simulink library "breaker_lib"  (Simulink 8.1)
settings: Solver=ode45  StartTime=0.0  StopTime=10.0  RelTol=1e-3
values from neighbouring files (symbols this model uses):
  Ts = 100E-6    (= 0.0001)    [UnitTest_Breaker_init.m]
undefined symbols (not defined in the file): cb_mech_delay
libraries: powerlib x17, simulink x5, breaker_lib x4, powerlib_extras x2
settings Model: Creator=RE25624  LastModifiedBy=RE25624

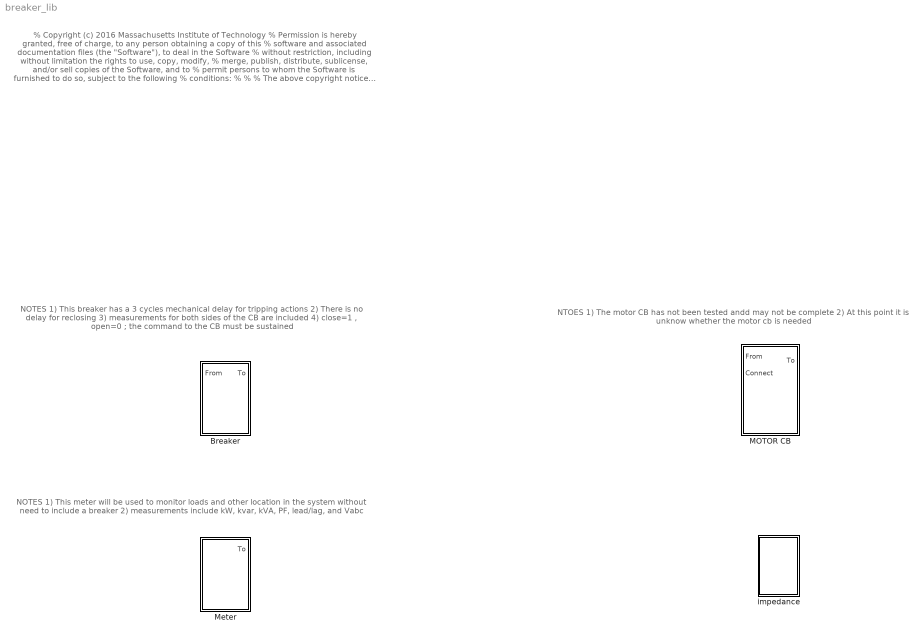
== system breaker_lib ==
  note: NTOES
      | 1) The motor CB has not been tested andd may not be complete
      | 2) At this point it is unknow whether the motor cb is needed
  note: NOTES
      | 1) This breaker has a 3 cycles mechanical delay for tripping actions
      | 2) There is no delay for reclosing
      | 3) measurements for both sides of the CB are included
      | 4) close=1 , open=0   ;  the command to the CB must be sustained
  note: NOTES
      | 1) This meter will be used to monitor loads and other location in the system without need to include a breaker
      | 2) measurements include kW, kvar, kVA, PF, lead/lag, and Vabc
  note: % Copyright (c) 2016 Massachusetts Institute of Technology
      | % Permission is hereby granted, free of charge, to any person obtaining a copy of this
      | % software and associated documentation files (the "Software"), to deal in the Software
      | % without restriction, including without limitation the rights to use, copy, modify,
      | % merge, publish, distribute, sublicense, and/or sell copies of the Software, and to
      | % permit persons to whom the Software is furnished to do so, subject to the following
      | % conditions:
      | %
      | %
      | % The above copyright notice and this permission notice shall be included in
      | % all copies or substantial portions of the Software.
      | %
      | % THE SOFTWARE IS PROVIDED "AS IS", WITHOUT WARRANTY OF ANY KIND, EXPRESS OR IMPLIED,
      | % INCLUDING BUT NOT LIMITED TO THE WARRANTIES OF MERCHANTABILITY, FITNESS FOR A
      | % PARTICULAR PURPOSE AND NONINFRINGEMENT. IN NO EVENT SHALL THE AUTHORS OR COPYRIGHT
      | % HOLDERS BE LIABLE FOR ANY CLAIM, DAMAGES OR OTHER LIABILITY, WHETHER IN AN ACTION
      | % OF CONTRACT, TORT OR OTHERWISE, ARISING FROM, OUT OF OR IN CONNECTION WITH THE
      | % SOFTWARE OR THE USE OR OTHER DEALINGS IN THE SOFTWARE.
      | %
      | %
      | %%
  Breaker : Subsystem  mask(Breaker){Ts=Ts, mech_delay=cb_mech_delay}
      mask prompts: Ts "Sampling Time [Sec]"; mech_delay "Open/Close Mechanical Delay [Sec]"
      mask help:
      | This block simulates the open/close behavior of a breaker. The logic (1-closed; 0-open) of operation is provided via external relay-blocks.
      | The breaker model also facilitates the system measurements for all logic functions to operate.
      | The connectivity convention adopted for this block is as follows: ABC indicates the “entry-point” or line, and the abc indicates the “exit-point” or bus.
      |
      | Ts [s]: simulation time step
      | Breaker mechanical open/close delay [s]
      mask init:
      | mech_delay = floor(mech_delay/Ts);
  MOTOR CB : Subsystem  mask(Breaker){Ts=Ts}
      mask prompts: Ts "Sampling Time [Sec]"
      mask help:
      | This block simulates the open/close behavior of a breaker. The logic (1-closed; 0-open) of operation is provided via external relay-blocks.
      | The breaker model also facilitates the system measurements for all logic functions to operate.
      | The connectivity convention adopted for this block is as follows: ABC indicates the “entry-point” or line, and the abc indicates the “exit-point” or bus.
  Meter : Subsystem  mask(Breaker){Ts=Ts}
      mask prompts: Ts "Sampling Time [Sec]"
      mask help:
      | This block simulates the open/close behavior of a breaker. The logic (1-closed; 0-open) of operation is provided via external relay-blocks.
      | The breaker model also facilitates the system measurements for all logic functions to operate.
      | The connectivity convention adopted for this block is as follows: ABC indicates the “entry-point” or line, and the abc indicates the “exit-point” or bus.
  impedance : Subsystem  mask(1/0AWG cable){length=10, par_sets=1}
      mask prompts: length "Length [ft]"; par_sets "No. of parallel sets"
      mask help:
      | This block represents a 1/0AWG cable based on Table 4A-7  60 Hz impedance data for three-phase copper cable circuits, in approximate ohms per ft at 75 degrees C (b) Three-conductor cable
      |
      | Page 181 of the Red Book

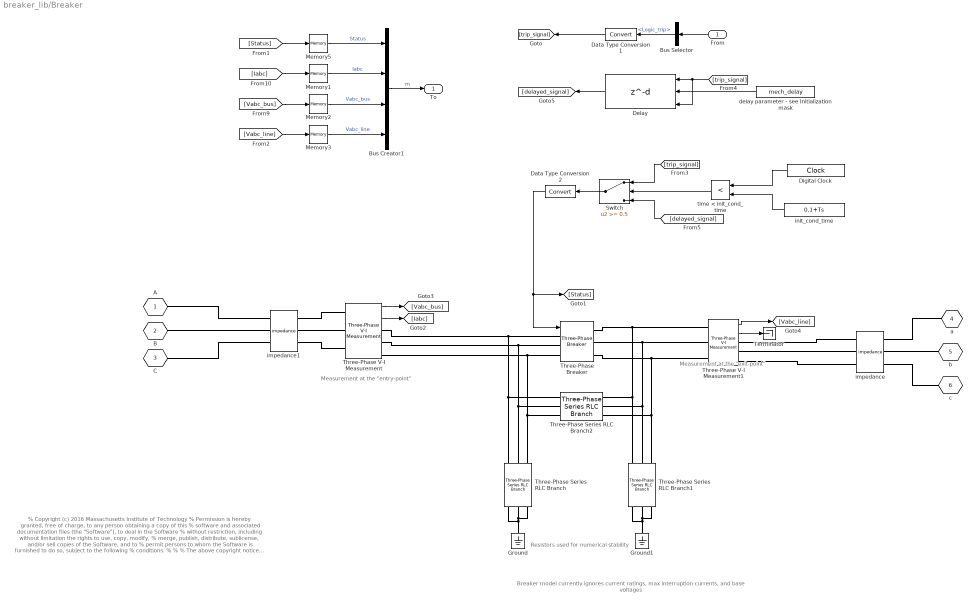
== system breaker_lib/Breaker ==
  note: % Copyright (c) 2016 Massachusetts Institute of Technology
      | % Permission is hereby granted, free of charge, to any person obtaining a copy of this
      | % software and associated documentation files (the "Software"), to deal in the Software
      | % without restriction, including without limitation the rights to use, copy, modify,
      | % merge, publish, distribute, sublicense, and/or sell copies of the Software, and to
      | % permit persons to whom the Software is furnished to do so, subject to the following
      | % conditions:
      | %
      | %
      | % The above copyright notice and this permission notice shall be included in
      | % all copies or substantial portions of the Software.
      | %
      | % THE SOFTWARE IS PROVIDED "AS IS", WITHOUT WARRANTY OF ANY KIND, EXPRESS OR IMPLIED,
      | % INCLUDING BUT NOT LIMITED TO THE WARRANTIES OF MERCHANTABILITY, FITNESS FOR A
      | % PARTICULAR PURPOSE AND NONINFRINGEMENT. IN NO EVENT SHALL THE AUTHORS OR COPYRIGHT
      | % HOLDERS BE LIABLE FOR ANY CLAIM, DAMAGES OR OTHER LIABILITY, WHETHER IN AN ACTION
      | % OF CONTRACT, TORT OR OTHERWISE, ARISING FROM, OUT OF OR IN CONNECTION WITH THE
      | % SOFTWARE OR THE USE OR OTHER DEALINGS IN THE SOFTWARE.
      | %
      | %
      | %%
  note: Measurement at the "exit-point"
  note: Measurement at the "entry-point"
  note: Resistors used for numerical stability
  note: Breaker model currently ignores current ratings, max interruption currents, and base voltages
  From : Inport
  Bus Creator1 : BusCreator
  Bus Selector : BusSelector  OutputSignals=Logic_trip
  Data Type Conversion1 : DataTypeConversion
  Data Type Conversion2 : DataTypeConversion
  Delay : Delay  DelayLengthSource=Input port  DelayLength=1  DelayLengthUpperLimit=5000  InitialConditionSource=Input port  InitialCondition=0
      settings: InputPortMap=u0,p1,p4
  Digital Clock : DigitalClock  SampleTime=Ts
  Ground : powerlib/Elements/Ground  LConnTagsString=a
  Ground1 : powerlib/Elements/Ground  LConnTagsString=a
  Memory{1..3,5} (4 alike) : Memory
  Switch : Switch  Threshold=0.5
  Terminator : Terminator
  Three-Phase Series RLC Branch : powerlib/Elements/Three-Phase Series RLC Branch  LConnTagsString=A|B|C  RConnTagsString=A|B|C  BranchType=R  Resistance=15E6  Inductance=1e-3  Capacitance=1e-6  Measurements=None
  Three-Phase Series RLC Branch1 : powerlib/Elements/Three-Phase Series RLC Branch  LConnTagsString=A|B|C  RConnTagsString=A|B|C  BranchType=R  Resistance=15E6  Inductance=1e-3  Capacitance=1e-6  Measurements=None
  Three-Phase Series RLC Branch2 : powerlib/Elements/Three-Phase Series RLC Branch  LConnTagsString=A|B|C  RConnTagsString=A|B|C  BranchType=R  Resistance=100E6  Inductance=1e-3  Capacitance=1e-6  Measurements=None
  Three-Phase V-I Measurement : powerlib/Measurements/Three-Phase V-I Measurement  VoltageMeasurement=phase-to-ground  SetLabelV=off  LabelV=Vabc  Vpu=off  VpuLL=off  CurrentMeasurement=yes  SetLabelI=off  LabelI=Iabc  Ipu=off  Pbase=100e6  Vbase=500e3  OutputType=Complex  PhasorSimulation=off  PSBequivalent=0
  Three-Phase V-I Measurement1 : powerlib/Measurements/Three-Phase V-I Measurement  VoltageMeasurement=phase-to-ground  SetLabelV=off  LabelV=Vabc  Vpu=off  VpuLL=off  CurrentMeasurement=yes  SetLabelI=off  LabelI=Iabc  Ipu=off  Pbase=100e6  Vbase=500e3  OutputType=Complex  PhasorSimulation=off  PSBequivalent=0
  Three-Phase Breaker : powerlib/Elements/Three-Phase Breaker  InitialState=open  SwitchA=on  SwitchB=on  SwitchC=on  SwitchTimes="[1/60  5/60]"  External=on  BreakerResistance=1e-4  SnubberResistance=1E15  SnubberCapacitance=inf  Measurements=None
  delay parameter - see Initialization mask : Constant  Value=mech_delay
  impedance : breaker_lib/impedance  length=10  par_sets=1
  impedance1 : breaker_lib/impedance  length=10  par_sets=1
  init_cond_time : Constant  Value=0.1+Ts
  time < init_cond_time : RelationalOperator  Operator=<  OutDataTypeStr=boolean
  A : PMIOPort  Tag=PMCPort  Port=1  Side=Left
  B : PMIOPort  Tag=PMCPort  Port=2  Side=Left
  C : PMIOPort  Tag=PMCPort  Port=3  Side=Left
  a : PMIOPort  Tag=PMCPort  Port=4  Side=Right
  b : PMIOPort  Tag=PMCPort  Port=5  Side=Right
  c : PMIOPort  Tag=PMCPort  Port=6  Side=Right
  To : Outport
  wires:
  [delayed_signal] -> Switch/3
  [trip_signal] -> Switch/1
  time < init_cond_time/1 -> Switch/2
  init_cond_time/1 -> time < init_cond_time/2
  Digital Clock/1 -> time < init_cond_time/1
  Delay/1 -> [delayed_signal]
  [trip_signal] -> Delay/1, Delay/3
  Data Type Conversion1/1 -> [trip_signal]
  Data Type Conversion2/1 -> Three-Phase Breaker/1, [Status]
  delay parameter - see Initialization mask/1 -> Delay/2
  Switch/1 -> Data Type Conversion2/1
  Bus Selector/1 -> Data Type Conversion1/1  "<Logic_trip>"
  Memory3/1 -> Bus Creator1/4  "Vabc_line"
  Memory2/1 -> Bus Creator1/3  "Vabc_bus"
  Memory1/1 -> Bus Creator1/2  "Iabc"
  Memory5/1 -> Bus Creator1/1  "Status"
  Three-Phase V-I Measurement1/2 -> Terminator/1
  [Vabc_line] -> Memory3/1
  Three-Phase V-I Measurement1/1 -> [Vabc_line]
  From/1 -> Bus Selector/1
  [Vabc_bus] -> Memory2/1
  [Iabc] -> Memory1/1
  [Status] -> Memory5/1
  Three-Phase V-I Measurement/2 -> [Iabc]
  Three-Phase V-I Measurement/1 -> [Vabc_bus]
  Bus Creator1/1 -> To/1  "m"
  connections:
  c/RConn1 -- impedance/RConn3
  b/RConn1 -- impedance/RConn2
  a/RConn1 -- impedance/RConn1
  impedance/LConn3 -- Three-Phase V-I Measurement1/RConn3
  impedance/LConn1 -- Three-Phase V-I Measurement1/RConn1
  impedance/LConn2 -- Three-Phase V-I Measurement1/RConn2
  C/RConn1 -- impedance1/LConn3
  B/RConn1 -- impedance1/LConn2
  A/RConn1 -- impedance1/LConn1
  impedance1/RConn1 -- Three-Phase V-I Measurement/LConn1
  impedance1/RConn3 -- Three-Phase V-I Measurement/LConn3
  impedance1/RConn2 -- Three-Phase V-I Measurement/LConn2
  Three-Phase Series RLC Branch1/RConn1 -- Ground1/LConn1 -- Three-Phase Series RLC Branch1/RConn3 -- Three-Phase Series RLC Branch1/RConn2
  Three-Phase Series RLC Branch/RConn1 -- Ground/LConn1 -- Three-Phase Series RLC Branch/RConn3 -- Three-Phase Series RLC Branch/RConn2
  Three-Phase Series RLC Branch2/LConn1 -- Three-Phase V-I Measurement/RConn1 -- Three-Phase Breaker/LConn1 -- Three-Phase Series RLC Branch/LConn1
  Three-Phase Series RLC Branch2/LConn2 -- Three-Phase V-I Measurement/RConn2 -- Three-Phase Breaker/LConn2 -- Three-Phase Series RLC Branch/LConn2
  Three-Phase Series RLC Branch2/LConn3 -- Three-Phase V-I Measurement/RConn3 -- Three-Phase Breaker/LConn3 -- Three-Phase Series RLC Branch/LConn3
  Three-Phase Series RLC Branch2/RConn1 -- Three-Phase V-I Measurement1/LConn1 -- Three-Phase Breaker/RConn1 -- Three-Phase Series RLC Branch1/LConn1
  Three-Phase Series RLC Branch2/RConn2 -- Three-Phase V-I Measurement1/LConn2 -- Three-Phase Breaker/RConn2 -- Three-Phase Series RLC Branch1/LConn2
  Three-Phase Series RLC Branch2/RConn3 -- Three-Phase V-I Measurement1/LConn3 -- Three-Phase Breaker/RConn3 -- Three-Phase Series RLC Branch1/LConn3

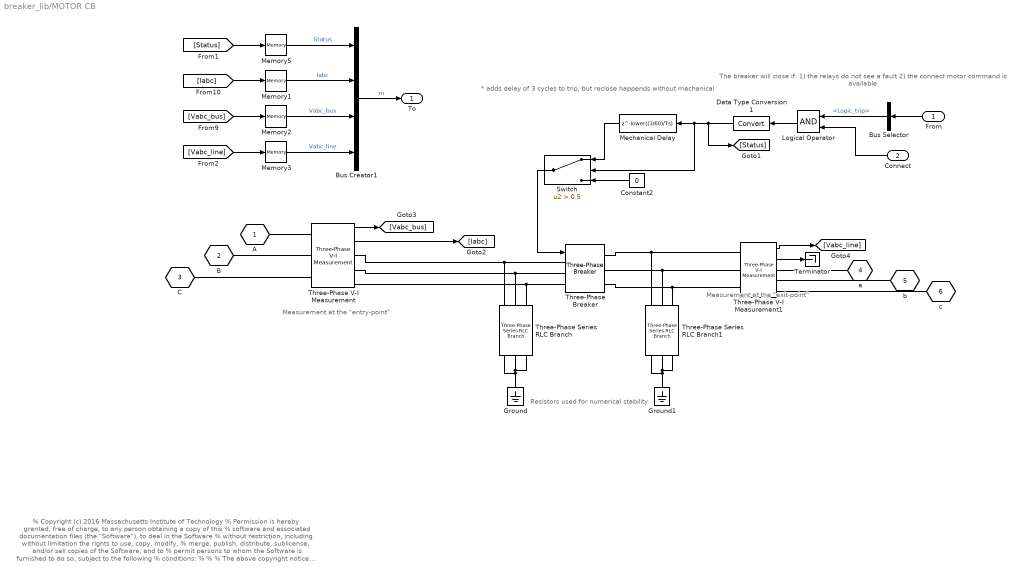
== system breaker_lib/MOTOR CB ==
  note: * adds delay of 3 cycles to trip, but reclose happends without mechanical
  note: Measurement at the "exit-point"
  note: Measurement at the "entry-point"
  note: Resistors used for numerical stability
  note: The breaker will close if:
      | 1) the relays do not see a fault
      | 2) the connect motor command is available
  note: % Copyright (c) 2016 Massachusetts Institute of Technology
      | % Permission is hereby granted, free of charge, to any person obtaining a copy of this
      | % software and associated documentation files (the "Software"), to deal in the Software
      | % without restriction, including without limitation the rights to use, copy, modify,
      | % merge, publish, distribute, sublicense, and/or sell copies of the Software, and to
      | % permit persons to whom the Software is furnished to do so, subject to the following
      | % conditions:
      | %
      | %
      | % The above copyright notice and this permission notice shall be included in
      | % all copies or substantial portions of the Software.
      | %
      | % THE SOFTWARE IS PROVIDED "AS IS", WITHOUT WARRANTY OF ANY KIND, EXPRESS OR IMPLIED,
      | % INCLUDING BUT NOT LIMITED TO THE WARRANTIES OF MERCHANTABILITY, FITNESS FOR A
      | % PARTICULAR PURPOSE AND NONINFRINGEMENT. IN NO EVENT SHALL THE AUTHORS OR COPYRIGHT
      | % HOLDERS BE LIABLE FOR ANY CLAIM, DAMAGES OR OTHER LIABILITY, WHETHER IN AN ACTION
      | % OF CONTRACT, TORT OR OTHERWISE, ARISING FROM, OUT OF OR IN CONNECTION WITH THE
      | % SOFTWARE OR THE USE OR OTHER DEALINGS IN THE SOFTWARE.
      | %
      | %
      | %%
  From : Inport
  Connect : Inport  Port=2
  Bus Creator1 : BusCreator
  Bus Selector : BusSelector  OutputSignals=Logic_trip
  Constant2 : Constant  Value=0
  Data Type Conversion1 : DataTypeConversion
  Ground : powerlib/Elements/Ground  LConnTagsString=a
  Ground1 : powerlib/Elements/Ground  LConnTagsString=a
  Logical Operator : Logic  AllPortsSameDT=off  OutDataTypeStr=boolean
  Mechanical Delay : Delay  DelayLength=lower((3/60)/Ts)  InitialCondition=1
  Memory{1..3,5} (4 alike) : Memory
  Switch : Switch  Criteria=u2 > Threshold  Threshold=0.5
  Terminator : Terminator
  Three-Phase Series RLC Branch : powerlib/Elements/Three-Phase Series RLC Branch  LConnTagsString=A|B|C  RConnTagsString=A|B|C  BranchType=R  Resistance=15E6  Inductance=1e-3  Capacitance=1e-6  Measurements=None
  Three-Phase Series RLC Branch1 : powerlib/Elements/Three-Phase Series RLC Branch  LConnTagsString=A|B|C  RConnTagsString=A|B|C  BranchType=R  Resistance=15E6  Inductance=1e-3  Capacitance=1e-6  Measurements=None
  Three-Phase V-I Measurement : powerlib/Measurements/Three-Phase V-I Measurement  VoltageMeasurement=phase-to-ground  SetLabelV=off  LabelV=Vabc  Vpu=off  VpuLL=off  CurrentMeasurement=yes  SetLabelI=off  LabelI=Iabc  Ipu=off  Pbase=100e6  Vbase=500e3  OutputType=Complex  PhasorSimulation=off  PSBequivalent=0
  Three-Phase V-I Measurement1 : powerlib/Measurements/Three-Phase V-I Measurement  VoltageMeasurement=phase-to-ground  SetLabelV=off  LabelV=Vabc  Vpu=off  VpuLL=off  CurrentMeasurement=yes  SetLabelI=off  LabelI=Iabc  Ipu=off  Pbase=100e6  Vbase=500e3  OutputType=Complex  PhasorSimulation=off  PSBequivalent=0
  Three-Phase Breaker : powerlib/Elements/Three-Phase Breaker  InitialState=open  SwitchA=on  SwitchB=on  SwitchC=on  SwitchTimes="[1/60  5/60]"  External=on  BreakerResistance=1e-4  SnubberResistance=1E15  SnubberCapacitance=inf  Measurements=None
  A : PMIOPort  Tag=PMCPort  Port=1  Side=Left
  B : PMIOPort  Tag=PMCPort  Port=2  Side=Left
  C : PMIOPort  Tag=PMCPort  Port=3  Side=Left
  a : PMIOPort  Tag=PMCPort  Port=4  Side=Right
  b : PMIOPort  Tag=PMCPort  Port=5  Side=Right
  c : PMIOPort  Tag=PMCPort  Port=6  Side=Right
  To : Outport
  wires:
  Constant2/1 -> Switch/3
  Mechanical Delay/1 -> Switch/1
  Switch/1 -> Three-Phase Breaker/1
  Memory3/1 -> Bus Creator1/4  "Vabc_line"
  Memory2/1 -> Bus Creator1/3  "Vabc_bus"
  Memory1/1 -> Bus Creator1/2  "Iabc"
  Memory5/1 -> Bus Creator1/1  "Status"
  Three-Phase V-I Measurement1/2 -> Terminator/1
  [Vabc_line] -> Memory3/1
  Three-Phase V-I Measurement1/1 -> [Vabc_line]
  From/1 -> Bus Selector/1
  [Vabc_bus] -> Memory2/1
  [Iabc] -> Memory1/1
  [Status] -> Memory5/1
  Data Type Conversion1/1 -> Switch/2, Mechanical Delay/1, [Status]
  Three-Phase V-I Measurement/2 -> [Iabc]
  Three-Phase V-I Measurement/1 -> [Vabc_bus]
  Bus Creator1/1 -> To/1  "m"
  Logical Operator/1 -> Data Type Conversion1/1
  Bus Selector/1 -> Logical Operator/1  "<Logic_trip>"
  Connect/1 -> Logical Operator/2
  connections:
  Three-Phase Series RLC Branch1/RConn1 -- Ground1/LConn1 -- Three-Phase Series RLC Branch1/RConn3 -- Three-Phase Series RLC Branch1/RConn2
  Three-Phase Series RLC Branch/RConn1 -- Ground/LConn1 -- Three-Phase Series RLC Branch/RConn3 -- Three-Phase Series RLC Branch/RConn2
  Three-Phase Series RLC Branch/LConn1 -- Three-Phase V-I Measurement/RConn1 -- Three-Phase Breaker/LConn1
  Three-Phase Series RLC Branch/LConn2 -- Three-Phase V-I Measurement/RConn2 -- Three-Phase Breaker/LConn2
  Three-Phase Series RLC Branch/LConn3 -- Three-Phase Breaker/LConn3 -- Three-Phase V-I Measurement/RConn3
  Three-Phase Series RLC Branch1/LConn1 -- Three-Phase V-I Measurement1/LConn1 -- Three-Phase Breaker/RConn1
  Three-Phase Series RLC Branch1/LConn2 -- Three-Phase V-I Measurement1/LConn2 -- Three-Phase Breaker/RConn2
  Three-Phase Series RLC Branch1/LConn3 -- Three-Phase V-I Measurement1/LConn3 -- Three-Phase Breaker/RConn3
  Three-Phase V-I Measurement/LConn1 -- A/RConn1
  B/RConn1 -- Three-Phase V-I Measurement/LConn2
  C/RConn1 -- Three-Phase V-I Measurement/LConn3
  a/RConn1 -- Three-Phase V-I Measurement1/RConn1
  b/RConn1 -- Three-Phase V-I Measurement1/RConn2
  c/RConn1 -- Three-Phase V-I Measurement1/RConn3

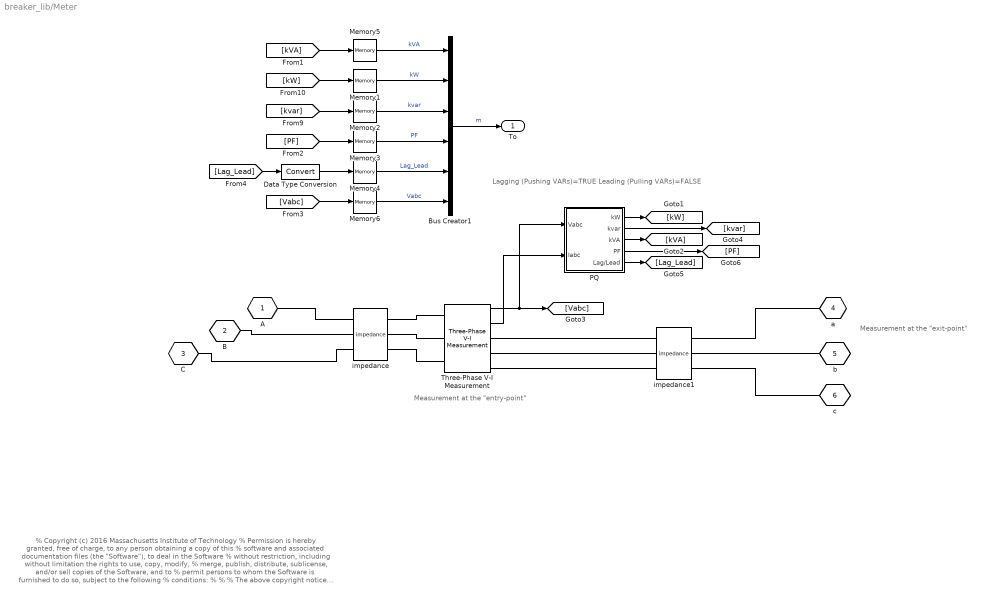
== system breaker_lib/Meter ==
  note: Lagging (Pushing VARs)=TRUE
      | Leading (Pulling VARs)=FALSE
  note: Measurement at the "entry-point"
  note: Measurement at the "exit-point"
  note: % Copyright (c) 2016 Massachusetts Institute of Technology
      | % Permission is hereby granted, free of charge, to any person obtaining a copy of this
      | % software and associated documentation files (the "Software"), to deal in the Software
      | % without restriction, including without limitation the rights to use, copy, modify,
      | % merge, publish, distribute, sublicense, and/or sell copies of the Software, and to
      | % permit persons to whom the Software is furnished to do so, subject to the following
      | % conditions:
      | %
      | %
      | % The above copyright notice and this permission notice shall be included in
      | % all copies or substantial portions of the Software.
      | %
      | % THE SOFTWARE IS PROVIDED "AS IS", WITHOUT WARRANTY OF ANY KIND, EXPRESS OR IMPLIED,
      | % INCLUDING BUT NOT LIMITED TO THE WARRANTIES OF MERCHANTABILITY, FITNESS FOR A
      | % PARTICULAR PURPOSE AND NONINFRINGEMENT. IN NO EVENT SHALL THE AUTHORS OR COPYRIGHT
      | % HOLDERS BE LIABLE FOR ANY CLAIM, DAMAGES OR OTHER LIABILITY, WHETHER IN AN ACTION
      | % OF CONTRACT, TORT OR OTHERWISE, ARISING FROM, OUT OF OR IN CONNECTION WITH THE
      | % SOFTWARE OR THE USE OR OTHER DEALINGS IN THE SOFTWARE.
      | %
      | %
      | %%
  Bus Creator1 : BusCreator  Inputs=6
  Data Type Conversion : DataTypeConversion
  Memory{1..6} (6 alike) : Memory
  PQ : Subsystem
  Three-Phase V-I Measurement : powerlib/Measurements/Three-Phase V-I Measurement  VoltageMeasurement=phase-to-ground  SetLabelV=off  LabelV=Vabc  Vpu=off  VpuLL=off  CurrentMeasurement=yes  SetLabelI=off  LabelI=Iabc  Ipu=off  Pbase=100e6  Vbase=500e3  OutputType=Complex  PhasorSimulation=off  PSBequivalent=0
  impedance : breaker_lib/impedance  length=10  par_sets=1
  impedance1 : breaker_lib/impedance  length=10  par_sets=1
  A : PMIOPort  Tag=PMCPort  Port=1  Side=Left
  B : PMIOPort  Tag=PMCPort  Port=2  Side=Left
  C : PMIOPort  Tag=PMCPort  Port=3  Side=Left
  a : PMIOPort  Tag=PMCPort  Port=4  Side=Right
  b : PMIOPort  Tag=PMCPort  Port=5  Side=Right
  c : PMIOPort  Tag=PMCPort  Port=6  Side=Right
  To : Outport
  wires:
  Bus Creator1/1 -> To/1  "m"
  Three-Phase V-I Measurement/1 -> PQ/1(Vabc), [Vabc]
  Three-Phase V-I Measurement/2 -> PQ/2(Iabc)
  [kVA] -> Memory5/1
  [kW] -> Memory1/1
  [kvar] -> Memory2/1
  [PF] -> Memory3/1
  Memory5/1 -> Bus Creator1/1  "kVA"
  Memory1/1 -> Bus Creator1/2  "kW"
  Memory2/1 -> Bus Creator1/3  "kvar"
  Memory3/1 -> Bus Creator1/4  "PF"
  PQ/2(kvar) -> [kvar]
  PQ/1(kW) -> [kW]
  PQ/3(kVA) -> [kVA]
  PQ/4(PF) -> [PF]
  PQ/5(Lag/Lead) -> [Lag_Lead]
  [Lag_Lead] -> Data Type Conversion/1
  [Vabc] -> Memory6/1
  Memory4/1 -> Bus Creator1/5  "Lag_Lead"
  Memory6/1 -> Bus Creator1/6  "Vabc"
  Data Type Conversion/1 -> Memory4/1
  connections:
  impedance/RConn1 -- Three-Phase V-I Measurement/LConn1
  impedance/RConn2 -- Three-Phase V-I Measurement/LConn2
  impedance/RConn3 -- Three-Phase V-I Measurement/LConn3
  A/RConn1 -- impedance/LConn1
  B/RConn1 -- impedance/LConn2
  C/RConn1 -- impedance/LConn3
  impedance1/LConn2 -- Three-Phase V-I Measurement/RConn2
  impedance1/LConn3 -- Three-Phase V-I Measurement/RConn3
  impedance1/LConn1 -- Three-Phase V-I Measurement/RConn1
  b/RConn1 -- impedance1/RConn2
  c/RConn1 -- impedance1/RConn3
  a/RConn1 -- impedance1/RConn1

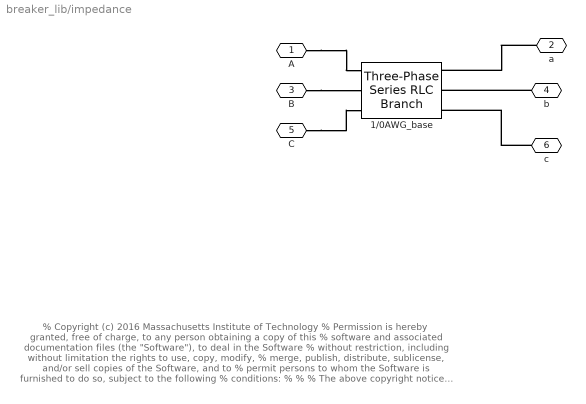
== system breaker_lib/impedance ==
  note: % Copyright (c) 2016 Massachusetts Institute of Technology
      | % Permission is hereby granted, free of charge, to any person obtaining a copy of this
      | % software and associated documentation files (the "Software"), to deal in the Software
      | % without restriction, including without limitation the rights to use, copy, modify,
      | % merge, publish, distribute, sublicense, and/or sell copies of the Software, and to
      | % permit persons to whom the Software is furnished to do so, subject to the following
      | % conditions:
      | %
      | %
      | % The above copyright notice and this permission notice shall be included in
      | % all copies or substantial portions of the Software.
      | %
      | % THE SOFTWARE IS PROVIDED "AS IS", WITHOUT WARRANTY OF ANY KIND, EXPRESS OR IMPLIED,
      | % INCLUDING BUT NOT LIMITED TO THE WARRANTIES OF MERCHANTABILITY, FITNESS FOR A
      | % PARTICULAR PURPOSE AND NONINFRINGEMENT. IN NO EVENT SHALL THE AUTHORS OR COPYRIGHT
      | % HOLDERS BE LIABLE FOR ANY CLAIM, DAMAGES OR OTHER LIABILITY, WHETHER IN AN ACTION
      | % OF CONTRACT, TORT OR OTHERWISE, ARISING FROM, OUT OF OR IN CONNECTION WITH THE
      | % SOFTWARE OR THE USE OR OTHER DEALINGS IN THE SOFTWARE.
      | %
      | %
      | %%
  1/0AWG_base : powerlib/Elements/Three-Phase Series RLC Branch  LConnTagsString=A|B|C  RConnTagsString=A|B|C  BranchType=RL  Resistance=0.000128*length/par_sets  Inductance=1.0982e-007*length/par_sets  Capacitance=0  Measurements=None
  A : PMIOPort  Port=1  Side=Left
  a : PMIOPort  Port=2  Side=Right
  B : PMIOPort  Port=3  Side=Left
  b : PMIOPort  Port=4  Side=Right
  C : PMIOPort  Port=5  Side=Left
  c : PMIOPort  Port=6  Side=Right
  connections:
  c/RConn1 -- 1/0AWG_base/RConn3
  C/RConn1 -- 1/0AWG_base/LConn3
  b/RConn1 -- 1/0AWG_base/RConn2
  B/RConn1 -- 1/0AWG_base/LConn2
  a/RConn1 -- 1/0AWG_base/RConn1
  A/RConn1 -- 1/0AWG_base/LConn1

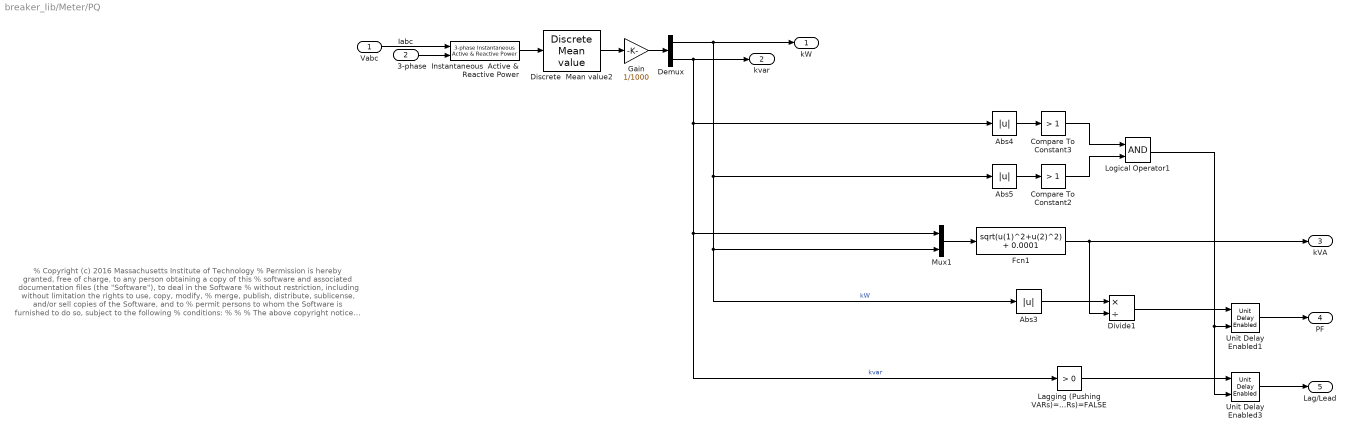
== system breaker_lib/Meter/PQ ==
  note: % Copyright (c) 2016 Massachusetts Institute of Technology
      | % Permission is hereby granted, free of charge, to any person obtaining a copy of this
      | % software and associated documentation files (the "Software"), to deal in the Software
      | % without restriction, including without limitation the rights to use, copy, modify,
      | % merge, publish, distribute, sublicense, and/or sell copies of the Software, and to
      | % permit persons to whom the Software is furnished to do so, subject to the following
      | % conditions:
      | %
      | %
      | % The above copyright notice and this permission notice shall be included in
      | % all copies or substantial portions of the Software.
      | %
      | % THE SOFTWARE IS PROVIDED "AS IS", WITHOUT WARRANTY OF ANY KIND, EXPRESS OR IMPLIED,
      | % INCLUDING BUT NOT LIMITED TO THE WARRANTIES OF MERCHANTABILITY, FITNESS FOR A
      | % PARTICULAR PURPOSE AND NONINFRINGEMENT. IN NO EVENT SHALL THE AUTHORS OR COPYRIGHT
      | % HOLDERS BE LIABLE FOR ANY CLAIM, DAMAGES OR OTHER LIABILITY, WHETHER IN AN ACTION
      | % OF CONTRACT, TORT OR OTHERWISE, ARISING FROM, OUT OF OR IN CONNECTION WITH THE
      | % SOFTWARE OR THE USE OR OTHER DEALINGS IN THE SOFTWARE.
      | %
      | %
      | %%
  Vabc : Inport
  Iabc : Inport  Port=2
  3-phase  Instantaneous  Active & Reactive Power : powerlib_extras/Measurements/3-phase  Instantaneous  Active & Reactive Power
  Abs3 : Abs
  Abs4 : Abs
  Abs5 : Abs
  Compare To Constant2 : simulink/Logic and Bit Operations/Compare To Constant  relop=>  const=1  OutDataTypeStr=uint8
  Compare To Constant3 : simulink/Logic and Bit Operations/Compare To Constant  relop=>  const=1  OutDataTypeStr=uint8
  Demux : Demux  Outputs=2
  Discrete  Mean value2 : powerlib_extras/Discrete Measurements/Discrete  Mean value  Freq=60  Vinit=0  Ts=Ts
  Divide1 : Product  Inputs=*/
  Fcn1 : Fcn  Expr=sqrt(u(1)^2+u(2)^2) + 0.0001
  Gain : Gain  Gain=1/1000
  Lagging (Pushing VARs)=TRUE Leading (Pulling VARs)=FALSE : simulink/Logic and Bit Operations/Compare To Constant  relop=>  const=0  OutDataTypeStr=boolean
  Logical Operator1 : Logic  AllPortsSameDT=off  OutDataTypeStr=boolean
  Mux1 : Mux  Inputs=2
  Unit Delay Enabled1 : simulink/Additional Math & Discrete/Additional Discrete/Unit Delay Enabled  vinit=1  tsamp=-1
  Unit Delay Enabled3 : simulink/Additional Math & Discrete/Additional Discrete/Unit Delay Enabled  vinit=1  tsamp=-1
  kW : Outport
  kvar : Outport  Port=2
  kVA : Outport  Port=3
  PF : Outport  Port=4
  Lag/Lead : Outport  Port=5
  wires:
  3-phase  Instantaneous  Active & Reactive Power/1 -> Discrete  Mean value2/1
  Discrete  Mean value2/1 -> Gain/1
  Vabc/1 -> 3-phase  Instantaneous  Active & Reactive Power/1
  Iabc/1 -> 3-phase  Instantaneous  Active & Reactive Power/2
  Demux/1 -> Abs3/1, Mux1/2, Abs5/1, kW/1  "kW"
  Demux/2 -> Mux1/1, Lagging (Pushing VARs)=TRUE Leading (Pulling VARs)=FALSE/1, Abs4/1, kvar/1  "kvar"
  Gain/1 -> Demux/1
  Logical Operator1/1 -> Unit Delay Enabled3/2, Unit Delay Enabled1/2
  Compare To Constant2/1 -> Logical Operator1/2
  Compare To Constant3/1 -> Logical Operator1/1
  Abs4/1 -> Compare To Constant3/1
  Abs5/1 -> Compare To Constant2/1
  Unit Delay Enabled3/1 -> Lag/Lead/1
  Lagging (Pushing VARs)=TRUE Leading (Pulling VARs)=FALSE/1 -> Unit Delay Enabled3/1
  Unit Delay Enabled1/1 -> PF/1
  Divide1/1 -> Unit Delay Enabled1/1
  Abs3/1 -> Divide1/1
  Mux1/1 -> Fcn1/1
  Fcn1/1 -> kVA/1, Divide1/2
